simulink model "sm_trackV_roller4_IdlerArm_i2u0r3_ptcld"  (R2026a)
settings: Solver=ode23t  StopTime=14  AbsTol=1e-3  EnableMultiTasking=on
PostLoadFcn:
  | set_param([bdroot '/Track FL'],'popup_sense_roller','Actuator Torque')
  | set_param([bdroot '/Track FR'],'popup_sense_roller','Actuator Torque')
  | set_param([bdroot '/Track RL'],'popup_sense_roller','Actuator Torque')
  | set_param([bdroot '/Track RR'],'popup_sense_roller','Actuator Torque')
StartFcn:
  | tic
StopFcn:
  | Elapsed_Sim_Time = toc;
  | disp(['Elapsed Sim Time = ' num2str(Elapsed_Sim_Time)]);
undefined symbols (not defined in the file): Scene, X, Y, Z
libraries: sm_lib x9, fl_lib x8, nesl_utility x5, sm_trackV_lib_chain_underc_elem x4, simulink x4, sm_rollerV_lib_lower_frame_idlerArm_i2u0l3 x4, sm_excv_chassis_lib x3, sm_rollerV_lib_terrain_contact_r5 x3
(part 1 of 2)
Description:
  | Belt Track (Four), Roller Contact Point Cloud
  | Copyright 2024-2026 The MathWorks, Inc.
settings Model: Creator=smiller  LastModifiedBy=smiller
settings DataIOCC: SignalLoggingName=logsout_sm_trackV_roller4_IdlerArm_i2u0r3_ptcld
settings DebuggingCC: SubsystemReferenceDiagnosticForUnitTest=warning
settings SimscapeCC: SimscapeNominalValues="[{\"value\":\"1\",\"unit\":\"A\"},{\"value\":\"1\",\"unit\":\"bar\"},{\"value\":\"1\",\"unit\":\"cm^2\"},{\"value\":\"1\",\"unit\":\"cm^3/s\"},{\"value\":\"1\",\"unit\":\"kJ/kg\"},{\"value\":\"1\",\"unit\":\"kW\"},{\"value\":\"1\",\"unit\":\"l\"},{\"value\":\"1\",\"unit\":\"N\"},{\"value\":\"1\",\"unit\":\"N*m\"},{\"value\":\"1\",\"unit\":\"V\"}]"  SimscapeLogSimulationStatistics=on  SimscapeLogName=simlog_sm_trackV_roller4_IdlerArm_i2u0r3_ptcld  SimscapeLogLimitData=off
settings DiagnosticsConfigSet: SimMechanicsUnconnectedFramePorts=none  SimMechanicsConflictingReferenceFrames=none
settings ExplorerConfigSet: InternalSimMechanicsExplorerSettings="<ExplorerConfiguration><canonicalview>default</canonicalview><AnimationSetting><BasePlaybackSpeed>1.0</BasePlaybackSpeed><PlaybackSpeedFactor>4.0</PlaybackSpeedFactor></AnimationSetting><TilePanel><TileInfo><Tiles Columns=\"2\" Count=\"3\" Rows=\"2\"><Column Weight=\"0.5\"/><Column Weight=\"0.5\"/><Row Weight=\"0.4992\"/><Row Weight=\"0.5008\"/><Tile Height=\"2\" Width=\"1\" X=\"0\" Y=\"0\"/><Tile Height=\"1\" Width=\"1\" X=\"1\" Y=\"0\"/><Tile Height=\"1\" Width=\"1\" X=\"1\" Y=\"1\"/></Tiles></TileInfo><SceneInfo><SceneViewer><BGColor><R>1</R><G>1</G><B>1</B></BGColor><Camera><DoPerspective>on</DoPerspective><Position><X>8</X><Y>-4.69999999999999929</Y><Z>3.49999999999999956</Z></Position><Center><X>7.32379042217759135</X><Y>-4.02379042217759064</Y><Z>3.20762829527726279</Z></Center><Up><X>0</X><Y>0</Y><Z>1</Z></Up><ViewLimDist>1</ViewLimDist><YLim>0.466307658154998583</YLim><XLim>0.48985854998100864</XLim></Camera></SceneViewer><SceneViewer><BGColor><R>1</R><G>1</G><B>1</B></BGColor><Camera><DoPerspective>on</DoPerspective><Position><X>3.92771833623717702e-16</X><Y>-4</Y><Z>1.10000000000000053</Z></Position><Center><X>1.70727228698686394e-16</X><Y>-3</Y><Z>1.10000000000000053</Z></Center><Up><X>0</X><Y>0</Y><Z>1</Z></Up><ViewLimDist>1</ViewLimDist><YLim>0.466307658154998583</YLim><XLim>0.996493077701092966</XLim></Camera></SceneViewer><SceneViewer><BGColor><R>1</R><G>1</G><B>1</B></BGColor><Camera><DoPerspective>on</DoPerspective><Position><X>2.00000000000000089</X><Y>-2.52493193448249121e-16</Y><Z>9</Z></Position><Center><X>2.00000000000000089</X><Y>-2.52493193448249121e-16</Y><Z>8</Z></Center><Up><X>0</X><Y>1</Y><Z>0</Z></Up><ViewLimDist>1</ViewLimDist><YLim>0.466307658154998583</YLim><XLim>0.993092077435901444</XLim></Camera></SceneViewer></SceneInfo></TilePanel><MechEditorPanel><Cameras><Camera><Id>Camera1</Id><Value><Name>Track_CtrRear_AimFront</Name><NativeCamera><PositionTrackingFeature>Chassis.Camera_Frames.CamF_CtrRear_AimLF.R</PositionTrackingFeature><CenterTrackingFeature>Config.World_Frame.W</CenterTrackingFeature><UpVectorTrackingFeature>Config.World_Frame.W</UpVectorTrackingFeature><CenterTrackingOrigin>off</CenterTrackingOrigin><CenterTrackingDirection>+X</CenterTrackingDirection><UpVectorTrackingDirection>+Z</UpVectorTrackingDirection></NativeCamera></Value></Camera><Camera><Id>Camera2</Id><Value><Name>Track_Left_AimRight</Name><NativeCamera><PositionTrackingFeature>Chassis.Camera_Frames.CamF_Left_AimRight.R</PositionTrackingFeature><CenterTrackingFeature>Chassis.Camera_Frames.CamF_Left_AimRight.R</CenterTrackingFeature><UpVectorTrackingFeature>Config.World_Frame.W</UpVectorTrackingFeature><CenterTrackingOrigin>off</CenterTrackingOrigin><CenterTrackingDirection>+X</CenterTrackingDirection><UpVectorTrackingDirection>+Z</UpVectorTrackingDirection></NativeCamera></Value></Camera><Camera><Id>Camera3</Id><Value><Name>Track_Front_AimLR</Name><NativeCamera><PositionTrackingFeature>Chassis.Camera_Frames.CamF_Front_AimLR.R</PositionTrackingFeature><CenterTrackingFeature>Chassis.Camera_Frames.Transform_Front_AimLR.F</CenterTrackingFeature><UpVectorTrackingFeature>Config.World_Frame.W</UpVectorTrackingFeature><CenterTrackingOrigin>off</CenterTrackingOrigin><CenterTrackingDirection>+X</CenterTrackingDirection><UpVectorTrackingDirection>+Z</UpVectorTrackingDirection></NativeCamera></Value></Camera><Camera><Id>Camera4</Id><Value><Name>Track_Right_AimLeftTL</Name><NativeCamera><PositionTrackingFeature>Chassis.Camera_Frames.CamF_Right_AimLeftTL.R</PositionTrackingFeature><CenterTrackingFeature>Chassis.Camera_Frames.CamF_Right_AimLeftTL.R</CenterTrackingFeature><UpVectorTrackingFeature>Config.World_Frame.W</UpVectorTrackingFeature><CenterTrackingOrigin>off</CenterTrackingOrigin><CenterTrackingDirection>+X</CenterTrackingDirection><UpVectorTrackingDirection>+Z</UpVectorTrackingDirection></NativeCamera></Value></Camera><Camera><Id>Camera5</Id><Value><Name>Track_Right_AimLeftTR</Name><NativeCamera><PositionTrackingFeature>Chassis.Camera_Frames.CamF_Right_AimLeftTR.R</PositionTrackingFeature><CenterTrackingFeature>Chassis.Camera_Frames.CamF_Right_AimLeftTR.R</CenterTrackingFeature><UpVectorTrackingFeature>Config.World_Frame.W</UpVectorTrackingFeature><CenterTrackingOrigin>off</CenterTrackingOrigin><CenterTrackingDirection>+X</CenterTrackingDirection><UpVectorTrackingDirection>+Z</UpVectorTrackingDirection></NativeCamera></Value></Camera><Camera><Id>Camera6</Id><Value><Name>Track_FR_AimFront</Name><NativeCamera><PositionTrackingFeature>Chassis.Camera_Frames.CamF_FR_Aim_Front_R</PositionTrackingFeature><CenterTrackingFeature>Chassis.Camera_Frames.CamF_FR_Aim_Front_R</CenterTrackingFeature><UpVectorTrackingFeature>Config.W</UpVectorTrackingFeature><CenterTrackingOrigin>off</CenterTrackingOrigin><CenterTrackingDirection>+X</CenterTrackingDirection><UpVectorTrackingDirection>+Z</UpVectorTrackingDirection></NativeCamera></Value></Camera><Camera><Id>Camera7</Id><Value><Name>TrackIsoFR</Name><NativeCamera><PositionKeyframeSet><Keyframe><Time>0</Time><Value><X>7.6744465174951229</X><Y>-7.3378434494995588</Y><Z>0.83192924808838675</Z></Value></Keyframe><Keyframe><Time>4.8580359639439301</Time><Value><X>7.6744465174951229</X><Y>-7.3378434494995588</Y><Z>0.83192924808838675</Z></Value></Keyframe><Keyframe><Time>7.0422197385672698</Time><Value><X>8.4041500304882533</X><Y>-6.0478565656515233</Y><Z>1.2378387423585568</Z></Value></Keyframe><Keyframe><Time>12.78196840006439</Time><Value><X>20.29732183415512</X><Y>-9.1045432763174095</Y><Z>1.6217023498793322</Z></Value></Keyframe></PositionKeyframeSet><CenterKeyframeSet><Keyframe><Time>0</Time><Value><X>-3.9707986865367024</X><Y>13.1242688081241</Y><Z>1.8580696339996621</Z></Value></Keyframe><Keyframe><Time>4.8580359639439301</Time><Value><X>4.507312599752261</X><Y>-1.7728039312810333</Y><Z>1.1110065851169071</Z></Value></Keyframe><Keyframe><Time>7.0422197385672698</Time><Value><X>6.9754199629584264</X><Y>-2.3648388994835718</Y><Z>1.2924635728623486</Z></Value></Keyframe><Keyframe><Time>12.78196840006439</Time><Value><X>16.536524754348189</X><Y>-2.4963653739311518</Y><Z>1.9530913158644347</Z></Value></Keyframe></CenterKeyframeSet><UpVectorKeyframeSet><Keyframe><Time>0</Time><Value><X>0.036204453435340365</X><Y>-0.029489201528742272</Y><Z>0.99890921736894867</Z></Value></Keyframe><Keyframe><Time>4.8580359639439301</Time><Value><X>0.036204453435340372</X><Y>-0.029489201528742279</Y><Z>0.99890921736894867</Z></Value></Keyframe><Keyframe><Time>7.0422197385672698</Time><Value><X>0.015774113925201387</X><Y>-0.0087099802030477149</Y><Z>0.99983764360756966</Z></Value></Keyframe><Keyframe><Time>12.78196840006439</Time><Value><X>0.036204453435340372</X><Y>-0.029489201528742286</Y><Z>0.99890921736894867</Z></Value></Keyframe></UpVectorKeyframeSet></NativeCamera></Value></Camera><Camera><Id>Camera8</Id><Value><Name>Track_IsoFR_Big</Name><NativeCamera><PositionTrackingFeature>Chassis.Camera_Frames.CamF_FR_AimCtr_Big.R</PositionTrackingFeature><CenterTrackingFeature>Chassis.Camera_Frames.CamF_FR_AimCtr_Big.R</CenterTrackingFeature><UpVectorTrackingFeature>Config.W.frame</UpVectorTrackingFeature><CenterTrackingOrigin>off</CenterTrackingOrigin><CenterTrackingDirection>+X</CenterTrackingDirection><UpVectorTrackingDirection>+Z</UpVectorTrackingDirection></NativeCamera></Value></Camera><Camera><Id>Camera9</Id><Value><Name>Track_Top_FixO</Name><NativeCamera><PositionTrackingFeature>Chassis.Camera_Frames.CamF_Top.R</PositionTrackingFeature><CenterTrackingFeature>Config.W</CenterTrackingFeature><UpVectorTrackingFeature>Config.W</UpVectorTrackingFeature><CenterTrackingOrigin>off</CenterTrackingOrigin><CenterTrackingDirection>-Z</CenterTrackingDirection><UpVectorTrackingDirection>+Y</UpVectorTrackingDirection></NativeCamera></Value></Camera><Camera><Id>Camera10</Id><Value><Name>Track_Terrain_Steer</Name><NativeCamera><PositionKeyframeSet><Keyframe><Time>1.954306185234983</Time><Value><X>6.8114446186923496</X><Y>-5.3171553607278206</Y><Z>2.3434891046120194</Z></Value></Keyframe><Keyframe><Time>3.2620190833091063</Time><Value><X>8.6993949048857981</X><Y>-5.3317331728841273</Y><Z>2.4343360662333233</Z></Value></Keyframe><Keyframe><Time>5.0400013056141875</Time><Value><X>10.892348868797249</X><Y>-5.3777629823446311</Y><Z>2.9548739629979583</Z></Value></Keyframe><Keyframe><Time>6.4399956757078574</Time><Value><X>12.590773161836934</X><Y>-5.02192612890686</Y><Z>3.4550574594673802</Z></Value></Keyframe><Keyframe><Time>8.274080048576554</Time><Value><X>14.467163111987707</X><Y>-3.5325878594240057</Y><Z>3.6687375492730663</Z></Value></Keyframe><Keyframe><Time>10.611771973115053</Time><Value><X>16.092056497155664</X><Y>-0.19034994331009364</Y><Z>3.5642210119966649</Z></Value></Keyframe><Keyframe><Time>12.781922870204893</Time><Value><X>16.438502065245114</X><Y>2.6045222313399137</Y><Z>3.7512090554216835</Z></Value></Keyframe><Keyframe><Time>14</Time><Value><X>15.821419267246833</X><Y>4.405488260701441</Y><Z>3.6561806172412985</Z></Value></Keyframe></PositionKeyframeSet><CenterKeyframeSet><Keyframe><Time>1.954306185234983</Time><Value><X>3.8269446610796178</X><Y>-1.4237791566024609</Y><Z>1.4146779468278596</Z></Value></Keyframe><Keyframe><Time>3.2620190833091063</Time><Value><X>5.6599243323637811</X><Y>-1.3666460332407318</Y><Z>1.4884174126531708</Z></Value></Keyframe><Keyframe><Time>5.0400013056141875</Time><Value><X>7.9655341663497534</X><Y>-1.5596390492794066</Y><Z>2.0440151286844124</Z></Value></Keyframe><Keyframe><Time>6.4399956757078574</Time><Value><X>8.8172775775206471</X><Y>-0.099279748271351664</Y><Z>2.280701670444107</Z></Value></Keyframe><Keyframe><Time>8.274080048576554</Time><Value><X>11.140862936281749</X><Y>0.80667772469433485</Y><Z>2.633554181468174</Z></Value></Keyframe><Keyframe><Time>10.611771973115053</Time><Value><X>12.246653975093967</X><Y>4.8261013508136488</Y><Z>2.3674869461938366</Z></Value></Keyframe><Keyframe><Time>12.781922870204893</Time><Value><X>13.419912109075547</X><Y>6.5423699352357101</Y><Z>2.8117886929204419</Z></Value></Keyframe><Keyframe><Time>14</Time><Value><X>13.045484539267546</X><Y>8.0267844133623925</Y><Z>2.7922773888123493</Z></Value></Keyframe></CenterKeyframeSet><UpVectorKeyframeSet><Keyframe><Time>1.954306185234983</Time><Value><X>-0.1264530356370476</X><Y>0.13743109156705063</Y><Z>0.98240639495519599</Z></Value></Keyframe><Keyframe><Time>3.2620190833091063</Time><Value><X>-0.1264530356370476</X><Y>0.13743109156705063</Y><Z>0.98240639495519599</Z></Value></Keyframe><Keyframe><Time>5.0400013056141875</Time><Value><X>-0.12645303563704768</X><Y>0.13743109156705072</Y><Z>0.98240639495519599</Z></Value></Keyframe><Keyframe><Time>6.4399956757078574</Time><Value><X>-0.12645303563704768</X><Y>0.13743109156705072</Y><Z>0.98240639495519599</Z></Value></Keyframe><Keyframe><Time>8.274080048576554</Time><Value><X>-0.12645303563704768</X><Y>0.13743109156705069</Y><Z>0.98240639495519611</Z></Value></Keyframe><Keyframe><Time>10.611771973115053</Time><Value><X>-0.12645303563704768</X><Y>0.13743109156705069</Y><Z>0.98240639495519599</Z></Value></Keyframe><Keyframe><Time>12.781922870204893</Time><Value><X>-0.12645303563704771</X><Y>0.13743109156705072</Y><Z>0.98240639495519599</Z></Value></Keyframe><Keyframe><Time>14</Time><Value><X>-0.12645303563704774</X><Y>0.13743109156705072</Y><Z>0.98240639495519588</Z></Value></Keyframe></UpVectorKeyframeSet></NativeCamera></Value></Camera></Cameras><GfxPanelCameraMap><MapElement CameraMLId=\"Camera8\" GfxPanelIndex=\"0\"/><MapElement CameraMLId=\"Camera5\" GfxPanelIndex=\"1\"/><MapElement CameraMLId=\"Camera9\" GfxPanelIndex=\"2\"/></GfxPanelCameraMap><VideoCreator><PlaybackSpeedRatio>0.5</PlaybackSpeedRatio><FrameRate>30</FrameRate><VideoFormat>MPEG-4</VideoFormat><FrameSize>auto</FrameSize></VideoCreator></MechEditorPanel></ExplorerConfiguration>"

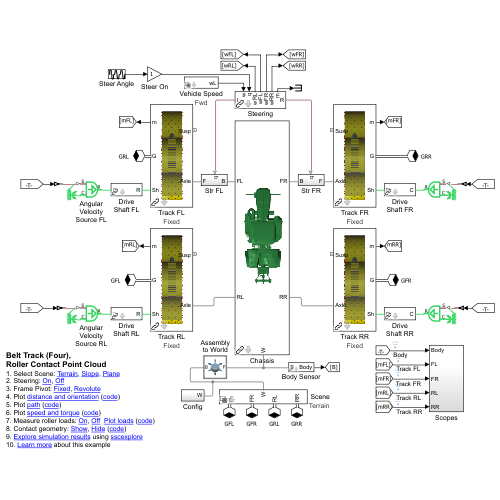
[thumbnail: Simulink's stored preview of the top-level diagram]
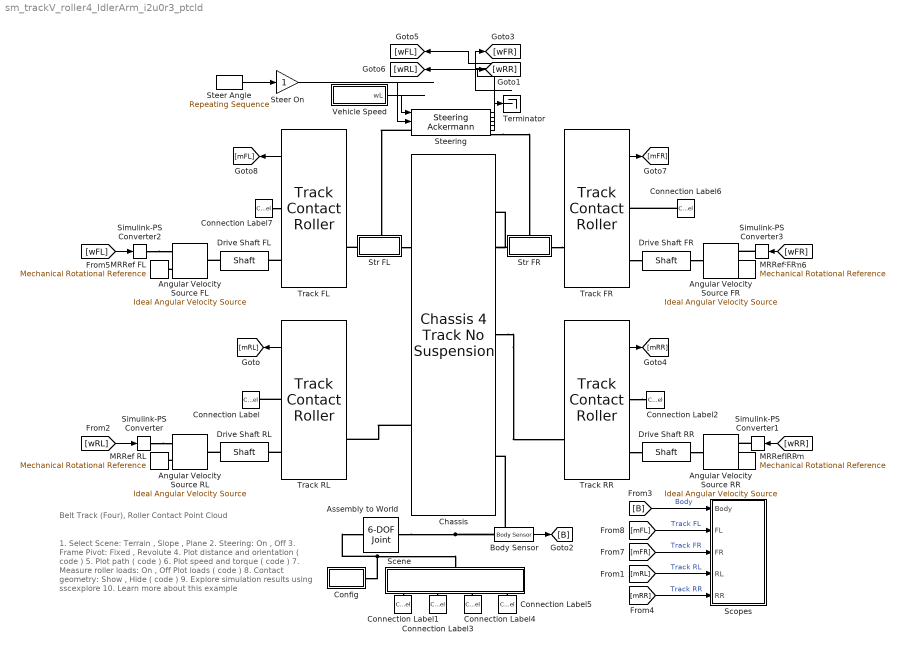
== system sm_trackV_roller4_IdlerArm_i2u0r3_ptcld ==
  note: 1. Select Scene: Terrain , Slope , Plane
      | 2. Steering: On , Off
      | 3. Frame Pivot: Fixed , Revolute
      | 4. Plot distance and orientation ( code )
      | 5. Plot path ( code )
      | 6. Plot speed and torque ( code )
      | 7. Measure roller loads: On , Off Plot loads ( code )
      | 8. Contact geometry: Show , Hide ( code )
      | 9. Explore simulation results using sscexplore
      | 10. Learn more about this example
  note: Belt Track (Four),
      | Roller Contact Point Cloud
  Angular Velocity Source FL : fl_lib/Mechanical/Mechanical Sources/Ideal Angular Velocity Source
  Angular Velocity Source FR : fl_lib/Mechanical/Mechanical Sources/Ideal Angular Velocity Source
  Angular Velocity Source RL : fl_lib/Mechanical/Mechanical Sources/Ideal Angular Velocity Source
  Angular Velocity Source RR : fl_lib/Mechanical/Mechanical Sources/Ideal Angular Velocity Source
  Assembly to World : sm_lib/Joints/6-DOF Joint  JointMode=Normal  CompositeWrenchDir=FollowerOnBase  CompositeWrenchFrame=BaseFrame  SenseConstraintForce=off  SenseConstraintTorque=off  SenseTotalForce=off  SenseTotalTorque=off  PxPositionTargetSpecify=on  PxPositionTargetPriority=High  PxPositionTargetValue=0  PxPositionTargetValueUnits=m  PxVelocityTargetSpecify=off  PxVelocityTargetPriority=High  PxVelocityTargetValue=0  PxVelocityTargetValueUnits=m/s  PxEquilibriumPosition=0  PxEquilibriumPositionUnits=m  PxSpringStiffness=0  PxSpringStiffnessUnits=N/m  PxDampingCoefficient=0  PxDampingCoefficientUnits=N/(m/s)  PxLowerLimitSpecify=off  PxLowerLimitBound=-1  PxLowerLimitBoundUnits=m  PxLowerLimitStiffness=1e6  PxLowerLimitStiffnessUnits=N/m  PxLowerLimitDamping=1e3  PxLowerLimitDampingUnits=N/(m/s)  PxLowerLimitTransitionRegionWidth=1e-4  PxLowerLimitTransitionRegionWidthUnits=m  PxUpperLimitSpecify=off  PxUpperLimitBound=1  PxUpperLimitBoundUnits=m  PxUpperLimitStiffness=1e6  PxUpperLimitStiffnessUnits=N/m  PxUpperLimitDamping=1e3  PxUpperLimitDampingUnits=N/(m/s)  PxUpperLimitTransitionRegionWidth=1e-4  PxUpperLimitTransitionRegionWidthUnits=m  PxTorqueActuationMode=NoTorque  PxMotionActuationMode=ComputedMotion  PxSensePosition=off  PxSenseVelocity=off  PxSenseAcceleration=off  PxSenseTorqueForce=off  PxSenseLowerLimitTorqueForce=off  PxSenseUpperLimitTorqueForce=off  PyPositionTargetSpecify=on  PyPositionTargetPriority=High  PyPositionTargetValue=0  PyPositionTargetValueUnits=m  PyVelocityTargetSpecify=off  PyVelocityTargetPriority=High  PyVelocityTargetValue=0  PyVelocityTargetValueUnits=m/s  PyEquilibriumPosition=0  PyEquilibriumPositionUnits=m  PySpringStiffness=0  PySpringStiffnessUnits=N/m  PyDampingCoefficient=0  PyDampingCoefficientUnits=N/(m/s)  PyLowerLimitSpecify=off  PyLowerLimitBound=-1  PyLowerLimitBoundUnits=m  PyLowerLimitStiffness=1e6  PyLowerLimitStiffnessUnits=N/m  PyLowerLimitDamping=1e3  PyLowerLimitDampingUnits=N/(m/s)  PyLowerLimitTransitionRegionWidth=1e-4  PyLowerLimitTransitionRegionWidthUnits=m  PyUpperLimitSpecify=off  PyUpperLimitBound=1  PyUpperLimitBoundUnits=m  PyUpperLimitStiffness=1e6  PyUpperLimitStiffnessUnits=N/m  PyUpperLimitDamping=1e3  PyUpperLimitDampingUnits=N/(m/s)  PyUpperLimitTransitionRegionWidth=1e-4  PyUpperLimitTransitionRegionWidthUnits=m  PyTorqueActuationMode=NoTorque  PyMotionActuationMode=ComputedMotion  PySensePosition=off  PySenseVelocity=off  PySenseAcceleration=off  PySenseTorqueForce=off  PySenseLowerLimitTorqueForce=off  PySenseUpperLimitTorqueForce=off  PzPositionTargetSpecify=on  PzPositionTargetPriority=High  PzPositionTargetValue=1.5  PzPositionTargetValueUnits=m  PzVelocityTargetSpecify=off  PzVelocityTargetPriority=High  PzVelocityTargetValue=0  PzVelocityTargetValueUnits=m/s  PzEquilibriumPosition=0  PzEquilibriumPositionUnits=m  PzSpringStiffness=0  PzSpringStiffnessUnits=N/m  PzDampingCoefficient=0  PzDampingCoefficientUnits=N/(m/s)  PzLowerLimitSpecify=off  PzLowerLimitBound=-1  PzLowerLimitBoundUnits=m  PzLowerLimitStiffness=1e6  PzLowerLimitStiffnessUnits=N/m  PzLowerLimitDamping=1e3  PzLowerLimitDampingUnits=N/(m/s)  PzLowerLimitTransitionRegionWidth=1e-4  PzLowerLimitTransitionRegionWidthUnits=m  PzUpperLimitSpecify=off  PzUpperLimitBound=1  PzUpperLimitBoundUnits=m  PzUpperLimitStiffness=1e6  PzUpperLimitStiffnessUnits=N/m  PzUpperLimitDamping=1e3  PzUpperLimitDampingUnits=N/(m/s)  PzUpperLimitTransitionRegionWidth=1e-4  PzUpperLimitTransitionRegionWidthUnits=m  PzTorqueActuationMode=NoTorque  PzMotionActuationMode=ComputedMotion  PzSensePosition=off  PzSenseVelocity=off  PzSenseAcceleration=off  PzSenseTorqueForce=off  PzSenseLowerLimitTorqueForce=off  PzSenseUpperLimitTorqueForce=off  SphPositionTargetSpecify=off  SphPositionTargetPriority=High  SphPositionTargetRotationMethod=StandardAxis  SphPositionTargetFollAlignAxisA=+X  SphPositionTargetBaseAlignAxisA=+Y  SphPositionTargetFollAlignAxisB=+Y  SphPositionTargetBaseAlignAxisB=+Z  SphPositionTargetRotationStandardAxis=+Z  SphPositionTargetRotationAngle=180  SphPositionTargetRotationAngleUnits=deg  SphPositionTargetRotationArbitraryAxis=[0 0 1]  SphPositionTargetRotationSequenceAxes=FollowerAxes  SphPositionTargetRotationSequence=XYX  SphPositionTargetRotationSequenceAngles=[0 0 0]  SphPositionTargetRotationSequenceAnglesUnits=deg  SphPositionTargetRotationMatrix=[1 0 0; 0 1 0; 0 0 1]  SphPositionTargetQuaternion=[1 0 0 0]  SphVelocityTargetSpecify=off  SphVelocityTargetPriority=High  SphVelocityTargetValue=[0 0 0]  SphVelocityTargetValueUnits=deg/s  SphVelocityTargetInFollowerFrame=on  SphEqPosRotationMethod=None  SphEqPosFollAlignAxisA=+X  SphEqPosBaseAlignAxisA=+Y  SphEqPosFollAlignAxisB=+Y  SphEqPosBaseAlignAxisB=+Z  SphEqPosRotationStandardAxis=+Z  SphEqPosRotationAngle=0.0  SphEqPosRotationAngleUnits=deg  SphEqPosRotationArbitraryAxis=[0 0 1]  SphEqPosRotationSequenceAxes=FollowerAxes  SphEqPosRotationSequence=XYX  SphEqPosRotationSequenceAngles=[0 0 0]  SphEqPosRotationSequenceAnglesUnits=deg  SphEqPosRotationMatrix=[1 0 0; 0 1 0; 0 0 1]  SphEqPosQuaternion=[1 0 0 0]  SphSpringStiffness=0  SphSpringStiffnessUnits=N*m/deg  SphDampingCoefficient=0  SphDampingCoefficientUnits=N*m/(deg/s)  SphLowerLimitSpecify=off  SphLowerLimitBound=15  SphLowerLimitBoundUnits=deg  SphLowerLimitStiffness=1e4  SphLowerLimitStiffnessUnits=N*m/deg  SphLowerLimitDamping=10  SphLowerLimitDampingUnits=N*m/(deg/s)  SphLowerLimitTransitionRegionWidth=0.1  SphLowerLimitTransitionRegionWidthUnits=deg  SphUpperLimitSpecify=off  SphUpperLimitBound=45  SphUpperLimitBoundUnits=deg  SphUpperLimitStiffness=1e4  SphUpperLimitStiffnessUnits=N*m/deg  SphUpperLimitDamping=10  SphUpperLimitDampingUnits=N*m/(deg/s)  SphUpperLimitTransitionRegionWidth=0.1  SphUpperLimitTransitionRegionWidthUnits=deg  SphTorqueActuationMode=NoTorque  SphActuateTorqueX=off  SphActuateTorqueY=off  SphActuateTorqueZ=off  SphActuateTorque=off  SphActuationFrame=BaseFrame  SphSensePosition=off  SphSenseVelocityX=off  SphSenseVelocityY=off  SphSenseVelocityZ=off  SphSenseVelocity=off  SphSenseAccelerationX=off  SphSenseAccelerationY=off  SphSenseAccelerationZ=off  SphSenseAcceleration=off  SphSenseLowerLimitTorqueMag=off  SphSenseUpperLimitTorqueMag=off  SphSensingFrame=BaseFrame
  Body Sensor : sm_excv_chassis_lib/Body Sensor  offset_body_sensor=[0 0 0]
  Chassis : sm_excv_chassis_lib/Chassis 4 Track No Suspension  popup_chassis_geo=CAD Shell
  Config : Subsystem
  Connection Label : ConnectionLabel  Label=GFL
  Connection Label1 : ConnectionLabel  Label=GFL
  Connection Label2 : ConnectionLabel  Label=GFR
  Connection Label3 : ConnectionLabel  Label=GFR
  Connection Label4 : ConnectionLabel  Label=GRL
  Connection Label5 : ConnectionLabel  Label=GRR
  Connection Label6 : ConnectionLabel  Label=GRR
  Connection Label7 : ConnectionLabel  Label=GRL
  Drive Shaft FL : sm_trackV_lib_chain_underc_elem/Shaft  k_shaft=Excv.Drive.Shaft.k  b_shaft=Excv.Drive.Shaft.b
  Drive Shaft FR : sm_trackV_lib_chain_underc_elem/Shaft  k_shaft=Excv.Drive.Shaft.k  b_shaft=Excv.Drive.Shaft.b
  Drive Shaft RL : sm_trackV_lib_chain_underc_elem/Shaft  k_shaft=Excv.Drive.Shaft.k  b_shaft=Excv.Drive.Shaft.b
  Drive Shaft RR : sm_trackV_lib_chain_underc_elem/Shaft  k_shaft=Excv.Drive.Shaft.k  b_shaft=Excv.Drive.Shaft.b
  MRRef FL : fl_lib/Mechanical/Rotational Elements/Mechanical Rotational Reference
  MRRef FR : fl_lib/Mechanical/Rotational Elements/Mechanical Rotational Reference
  MRRef RL : fl_lib/Mechanical/Rotational Elements/Mechanical Rotational Reference
  MRRef RR : fl_lib/Mechanical/Rotational Elements/Mechanical Rotational Reference
  Scene : Subsystem  Variant=on  VariantControlMode=label  VariantControl=Terrain  LabelModeActiveChoice=Terrain
      settings: AttributesFormatString=%<LabelModeActiveChoice>
      mask Display: disp(' ')
  Scopes : Subsystem
  Simulink-PS Converter{,1..3} (4 alike) : nesl_utility/Simulink-PS Converter  PhysicalDomain=network_engine_domain  SubClassName=ps_input  LeftPortType=input  RightPortType=output  PseudoPeriodic=off  Frequencies=[]  NoiseDistribution=none  NoiseParameters=[]  Unit=1  AffineConversion=off  FilteringAndDerivatives=provide  SimscapeFilterOrder=1  InputFilterTimeConstant=0.001  UdotUserProvided=0
  Steer Angle : simulink/Sources/Repeating Sequence  rep_seq_t="[0 3  5  14 16 18  20  29 31 36]"  rep_seq_y="[0 0 20 20  0   0 -20 -20  0   0]*pi/180"
  Steer On : Gain
  Steering : sm_excv_chassis_lib/Steering Ackermann  yTrack=Trac.Chassis.Front.TrackSepCtr  steerRatio=1  tcSteer=0.1  wheelbase=Trac.Chassis.AxleSeparation
  Str FL : Subsystem
      settings: PortSchema="{\"entries\":[{\"content\":{\"sides\":[{\"content\":{\"connectorIds\":[\"LConn1\"]},\"type\":\"ConnectorPlacement.EquallySpacedRectSide\",\"uuid\":\"c7c7e178-8ee1-427d-9e3f-0887a6c2686c\"},{\"content\":{\"connectorIds\":[\"RConn1\"],\"side\":\"RIGHT\"},\"type\":\"ConnectorPlacement.EquallySpacedRectSide\",\"uuid\":\"0bc250c9-893f-4ff8-8fb1-de52c2b7a8cd\"},{\"content\":{\"connectorIds\":[\"LConn2\"],\"side\":\"TOP\"},\"type\":\"ConnectorPlacement.EquallySpacedRectSide\",\"uuid\":\"31ffd3a3-da84-490a-ac6f-43ff5d5145cd\"}]},\"type\":\"ConnectorPlacement.EquallySpacedConnector\",\"uuid\":\"2f775820-965f-444f-9db7-4d7e95d78bbe\"}],\"packageUris\":[\"http://schema.mathworks.com/mf0/Connector/R2020b\"],\"version\":\"1.0\"}"
  Str FR : Subsystem
      settings: PortSchema="{\"entries\":[{\"content\":{\"sides\":[{\"content\":{\"connectorIds\":[\"LConn1\"]},\"type\":\"ConnectorPlacement.EquallySpacedRectSide\",\"uuid\":\"c7c7e178-8ee1-427d-9e3f-0887a6c2686c\"},{\"content\":{\"connectorIds\":[\"RConn1\"],\"side\":\"RIGHT\"},\"type\":\"ConnectorPlacement.EquallySpacedRectSide\",\"uuid\":\"0bc250c9-893f-4ff8-8fb1-de52c2b7a8cd\"},{\"content\":{\"connectorIds\":[\"LConn2\"],\"side\":\"TOP\"},\"type\":\"ConnectorPlacement.EquallySpacedRectSide\",\"uuid\":\"31ffd3a3-da84-490a-ac6f-43ff5d5145cd\"}]},\"type\":\"ConnectorPlacement.EquallySpacedConnector\",\"uuid\":\"2f775820-965f-444f-9db7-4d7e95d78bbe\"}],\"packageUris\":[\"http://schema.mathworks.com/mf0/Connector/R2020b\"],\"version\":\"1.0\"}"
  Terminator : Terminator
  Track FL : sm_rollerV_lib_lower_frame_idlerArm_i2u0l3/Track Contact Roller  sprk_wid_roll=Trac.Sprocket.Roller.wid  sprk_rad_roll=Trac.Sprocket.Roller.rad  sprk_clr=Trac.Sprocket.Roller.clr  sprk_opc=Trac.Sprocket.Roller.opc  sprk_rad_pitch=Trac.Sprocket.Spoke.pitch_rad  sprk_spoke_rad=Trac.Sprocket.Spoke.rad  sprk_spoke_num=Trac.Sprocket.nSpokes  sprk_spoke_len=Trac.Sprocket.Spoke.len  sprk_rim_spoke_xc=Trac.Sprocket.Rim.spoke_xc  sprk_rim_ir=Trac.Sprocket.Rim.rad_inner  sprk_rim_thk=Trac.Sprocket.Rim.thk  idlerR_rad=Trac.IdlerR.rad  idlerF_rad=Trac.IdlerF.rad  idlerR_total_len=Trac.IdlerR.len_total  idlerF_total_len=Trac.IdlerF.len_total  idlerR_avg_rho=Trac.IdlerR.rho_avg  idlerF_avg_rho=Trac.IdlerF.rho_avg  idlerR_clr=Trac.IdlerR.clr  idlerF_clr=Trac.IdlerF.clr  idlerR_opc=Trac.IdlerR.opc  idlerF_opc=Trac.IdlerF.opc  idlerR_contgeo_ptcld=Trac.IdlerR.ground_contact.ptcld.pts  idlerF_contgeo_ptcld=Trac.IdlerF.ground_contact.ptcld.pts  idlerR_contgeo_rad=Trac.IdlerR.ground_contact.ptcld.rad  idlerF_contgeo_rad=Trac.IdlerF.ground_contact.ptcld.rad  idlerR_contgeo_clr=Trac.IdlerR.belt_contact.clr  idlerF_contgeo_clr=Trac.IdlerF.belt_contact.clr  idlerR_contgeo_opc=Trac.IdlerR.belt_contact.opc  idlerF_contgeo_opc=Trac.IdlerF.belt_contact.opc  arm_idlerc=Trac.IdlerArm.Pivot_to_Idler  arm_tens_x=Trac.IdlerArm.Pivot_to_TensionerX  arm_tens_y=Trac.IdlerArm.Pivot_to_TensionerY  arm_wid=Trac.IdlerArm.wid  arm_thk=Trac.IdlerArm.thk  arm_rho=Trac.IdlerArm.rho  arm_clr=Trac.IdlerArm.clr  arm_opc=Trac.IdlerArm.opc  roller_lower_rad=Trac.Roller.Lower.rad  roller_lower_len=Trac.Roller.Lower.len  roller_lower_rho=Trac.Roller.Lower.rho  roller_lower_clr=Trac.Roller.Lower.clr  roller_lower_opc=Trac.Roller.Lower.opc  roller_lower_contgeo_ptcld=Trac.Roller.Lower.ground_contact.ptcld.pts  roller_lower_contgeo_rad=Trac.Roller.Lower.ground_contact.ptcld.rad  roller_lower_contgeo_clr=Trac.Roller.Lower.belt_contact.clr  roller_lower_contgeo_opc=Trac.Roller.Lower.belt_contact.opc  tensioner_cyl_len=Trac.IdlerF.Tensioner.cyl.len  tensioner_cyl_rad=Trac.IdlerF.Tensioner.cyl.rad  tensioner_cyl_rho=Trac.IdlerF.Tensioner.cyl.rho  tensioner_cyl_clr=Trac.IdlerF.Tensioner.cyl.clr  tensioner_cyl_opc=Trac.IdlerF.Tensioner.cyl.opc  tensioner_pist_len=Trac.IdlerF.Tensioner.piston.len  tensioner_pist_rad=Trac.IdlerF.Tensioner.piston.rad  tensioner_pist_rho=Trac.IdlerF.Tensioner.piston.rho  tensioner_pist_clr=Trac.IdlerF.Tensioner.piston.clr  tensioner_pist_opc=Trac.IdlerF.Tensioner.piston.opc  tensioner_br_len=Trac.IdlerF.Tensioner.bracket.len  tensioner_br_width=Trac.IdlerF.Tensioner.bracket.wid  tensioner_br_height=Trac.IdlerF.Tensioner.bracket.height  tensioner_br_thk=Trac.IdlerF.Tensioner.bracket.thk  tensioner_br_rho=Trac.IdlerF.Tensioner.bracket.rho  tensioner_br_clr=Trac.IdlerF.Tensioner.bracket.clr  tensioner_br_opc=Trac.IdlerF.Tensioner.bracket.opc  tensioner_eqpos=Trac.IdlerF.Tensioner.xeq  tensioner_x0=Trac.IdlerF.Tensioner.x0  tensioner_k=Trac.IdlerF.Tensioner.K  tensioner_b=Trac.IdlerF.Tensioner.B  popup_leftOrRight=Left  popup_trackFrame=Fixed  roller_lower_x=Trac.Frame.SprkOffLon.Lower  idlerFix_x=Trac.Frame.SprkOffLon.IdlerR  idlerArm_x=Trac.Frame.SprkOffLon.IdlerArm  tensionC_x=Trac.Frame.SprkOffLon.TensionC  frame_pivot_x=Trac.Frame.SprkOffLon.PivotFra  axle_x=Trac.Frame.SprkOffLon.Axle  roller_lower_y=Trac.Frame.SprkOffVer.Lower  idlerFix_y=Trac.Frame.SprkOffVer.IdlerR  tensionC_y=Trac.Frame.SprkOffVer.TensionC  frame_pivot_y=Trac.Frame.SprkOffVer.PivotFra  axle_y=Trac.Frame.SprkOffVer.Axle  idlerArm_y=Trac.Frame.SprkOffVer.IdlerArm  frame_mass=Trac.Frame.TrackFrame.Mass  frame_cg_offset=Trac.Frame.TrackFrame.CG  frame_moi=Trac.Frame.TrackFrame.MOI  frame_poi=Trac.Frame.TrackFrame.POI  frame_roller_cg_offset=Trac.Frame.SprkFrame.CG  frame_roller_mass=Trac.Frame.SprkFrame.Mass  frame_roller_moi=Trac.Frame.SprkFrame.MOI  frame_roller_poi=Trac.Frame.SprkFrame.POI  frame_susp_offset=Trac.Frame.SuspOffset  roller_frame_pivot_range=Trac.Frame.PivotFra.Range  roller_frame_pivot_k=Trac.Frame.PivotFra.LimitK  roller_frame_pivot_b=Trac.Frame.PivotFra.LimitB  roller_frame_pivot_tw=Trac.Frame.PivotFra.LimitTW  sprk_rolling_rad=Trac.Sprocket.ground_contact.rolling_radius  roller_lower_rolling_rad=Trac.Roller.Lower.ground_contact.rolling_radius  idlerF_rolling_rad=Trac.IdlerF.ground_contact.rolling_radius  idlerR_rolling_rad=Trac.IdlerR.ground_contact.rolling_radius  rolling_cyl_len=Trac.Belt.w  accent_vis_lext=1e-3  roller_lower_cyl_clr=Trac.Roller.Lower.clr  roller_lower_cyl_opc=Trac.Roller.Lower.opc  idlerR_rollvervis_clr=Trac.IdlerR.clr  idlerF_rollvervis_clr=Trac.IdlerF.clr  idlerR_rollervis_opc=Trac.IdlerR.opc  idlerF_rollervis_opc=Trac.IdlerF.opc  accMn=0.65  accMx=0.75  acc_clr=[0.8 0.8 0.8]  acc_opc=1  track_m=Trac.Vis.Track.m  track_cg_offset=Trac.Vis.Track.cg  track_moi=Trac.Vis.Track.moi  track_poi=Trac.Vis.Track.poi  track_xc=Trac.Vis.Track.track_xc  track_clr=Trac.Vis.Track.clr  track_opc=Trac.Vis.Track.opc  popup_sense_roller=Actuator Torque
      settings: AttributesFormatString=%<popup_trackFrame>
  Track FR : sm_rollerV_lib_lower_frame_idlerArm_i2u0l3/Track Contact Roller  sprk_wid_roll=Trac.Sprocket.Roller.wid  sprk_rad_roll=Trac.Sprocket.Roller.rad  sprk_clr=Trac.Sprocket.Roller.clr  sprk_opc=Trac.Sprocket.Roller.opc  sprk_rad_pitch=Trac.Sprocket.Spoke.pitch_rad  sprk_spoke_rad=Trac.Sprocket.Spoke.rad  sprk_spoke_num=Trac.Sprocket.nSpokes  sprk_spoke_len=Trac.Sprocket.Spoke.len  sprk_rim_spoke_xc=Trac.Sprocket.Rim.spoke_xc  sprk_rim_ir=Trac.Sprocket.Rim.rad_inner  sprk_rim_thk=Trac.Sprocket.Rim.thk  idlerR_rad=Trac.IdlerR.rad  idlerF_rad=Trac.IdlerF.rad  idlerR_total_len=Trac.IdlerR.len_total  idlerF_total_len=Trac.IdlerF.len_total  idlerR_avg_rho=Trac.IdlerR.rho_avg  idlerF_avg_rho=Trac.IdlerF.rho_avg  idlerR_clr=Trac.IdlerR.clr  idlerF_clr=Trac.IdlerF.clr  idlerR_opc=Trac.IdlerR.opc  idlerF_opc=Trac.IdlerF.opc  idlerR_contgeo_ptcld=Trac.IdlerR.ground_contact.ptcld.pts  idlerF_contgeo_ptcld=Trac.IdlerF.ground_contact.ptcld.pts  idlerR_contgeo_rad=Trac.IdlerR.ground_contact.ptcld.rad  idlerF_contgeo_rad=Trac.IdlerF.ground_contact.ptcld.rad  idlerR_contgeo_clr=Trac.IdlerR.belt_contact.clr  idlerF_contgeo_clr=Trac.IdlerF.belt_contact.clr  idlerR_contgeo_opc=Trac.IdlerR.belt_contact.opc  idlerF_contgeo_opc=Trac.IdlerF.belt_contact.opc  arm_idlerc=Trac.IdlerArm.Pivot_to_Idler  arm_tens_x=Trac.IdlerArm.Pivot_to_TensionerX  arm_tens_y=Trac.IdlerArm.Pivot_to_TensionerY  arm_wid=Trac.IdlerArm.wid  arm_thk=Trac.IdlerArm.thk  arm_rho=Trac.IdlerArm.rho  arm_clr=Trac.IdlerArm.clr  arm_opc=Trac.IdlerArm.opc  roller_lower_rad=Trac.Roller.Lower.rad  roller_lower_len=Trac.Roller.Lower.len  roller_lower_rho=Trac.Roller.Lower.rho  roller_lower_clr=Trac.Roller.Lower.clr  roller_lower_opc=Trac.Roller.Lower.opc  roller_lower_contgeo_ptcld=Trac.Roller.Lower.ground_contact.ptcld.pts  roller_lower_contgeo_rad=Trac.Roller.Lower.ground_contact.ptcld.rad  roller_lower_contgeo_clr=Trac.Roller.Lower.belt_contact.clr  roller_lower_contgeo_opc=Trac.Roller.Lower.belt_contact.opc  tensioner_cyl_len=Trac.IdlerF.Tensioner.cyl.len  tensioner_cyl_rad=Trac.IdlerF.Tensioner.cyl.rad  tensioner_cyl_rho=Trac.IdlerF.Tensioner.cyl.rho  tensioner_cyl_clr=Trac.IdlerF.Tensioner.cyl.clr  tensioner_cyl_opc=Trac.IdlerF.Tensioner.cyl.opc  tensioner_pist_len=Trac.IdlerF.Tensioner.piston.len  tensioner_pist_rad=Trac.IdlerF.Tensioner.piston.rad  tensioner_pist_rho=Trac.IdlerF.Tensioner.piston.rho  tensioner_pist_clr=Trac.IdlerF.Tensioner.piston.clr  tensioner_pist_opc=Trac.IdlerF.Tensioner.piston.opc  tensioner_br_len=Trac.IdlerF.Tensioner.bracket.len  tensioner_br_width=Trac.IdlerF.Tensioner.bracket.wid  tensioner_br_height=Trac.IdlerF.Tensioner.bracket.height  tensioner_br_thk=Trac.IdlerF.Tensioner.bracket.thk  tensioner_br_rho=Trac.IdlerF.Tensioner.bracket.rho  tensioner_br_clr=Trac.IdlerF.Tensioner.bracket.clr  tensioner_br_opc=Trac.IdlerF.Tensioner.bracket.opc  tensioner_eqpos=Trac.IdlerF.Tensioner.xeq  tensioner_x0=Trac.IdlerF.Tensioner.x0  tensioner_k=Trac.IdlerF.Tensioner.K  tensioner_b=Trac.IdlerF.Tensioner.B  popup_leftOrRight=Right  popup_trackFrame=Fixed  roller_lower_x=Trac.Frame.SprkOffLon.Lower  idlerFix_x=Trac.Frame.SprkOffLon.IdlerR  idlerArm_x=Trac.Frame.SprkOffLon.IdlerArm  tensionC_x=Trac.Frame.SprkOffLon.TensionC  frame_pivot_x=Trac.Frame.SprkOffLon.PivotFra  axle_x=Trac.Frame.SprkOffLon.Axle  roller_lower_y=Trac.Frame.SprkOffVer.Lower  idlerFix_y=Trac.Frame.SprkOffVer.IdlerR  tensionC_y=Trac.Frame.SprkOffVer.TensionC  frame_pivot_y=Trac.Frame.SprkOffVer.PivotFra  axle_y=Trac.Frame.SprkOffVer.Axle  idlerArm_y=Trac.Frame.SprkOffVer.IdlerArm  frame_mass=Trac.Frame.TrackFrame.Mass  frame_cg_offset=Trac.Frame.TrackFrame.CG  frame_moi=Trac.Frame.TrackFrame.MOI  frame_poi=Trac.Frame.TrackFrame.POI  frame_roller_cg_offset=Trac.Frame.SprkFrame.CG  frame_roller_mass=Trac.Frame.SprkFrame.Mass  frame_roller_moi=Trac.Frame.SprkFrame.MOI  frame_roller_poi=Trac.Frame.SprkFrame.POI  frame_susp_offset=Trac.Frame.SuspOffset  roller_frame_pivot_range=Trac.Frame.PivotFra.Range  roller_frame_pivot_k=Trac.Frame.PivotFra.LimitK  roller_frame_pivot_b=Trac.Frame.PivotFra.LimitB  roller_frame_pivot_tw=Trac.Frame.PivotFra.LimitTW  sprk_rolling_rad=Trac.Sprocket.ground_contact.rolling_radius  roller_lower_rolling_rad=Trac.Roller.Lower.ground_contact.rolling_radius  idlerF_rolling_rad=Trac.IdlerF.ground_contact.rolling_radius  idlerR_rolling_rad=Trac.IdlerR.ground_contact.rolling_radius  rolling_cyl_len=Trac.Belt.w  accent_vis_lext=1e-3  roller_lower_cyl_clr=Trac.Roller.Lower.clr  roller_lower_cyl_opc=Trac.Roller.Lower.opc  idlerR_rollvervis_clr=Trac.IdlerR.clr  idlerF_rollvervis_clr=Trac.IdlerF.clr  idlerR_rollervis_opc=Trac.IdlerR.opc  idlerF_rollervis_opc=Trac.IdlerF.opc  accMn=0.65  accMx=0.75  acc_clr=[0.8 0.8 0.8]  acc_opc=1  track_m=Trac.Vis.Track.m  track_cg_offset=Trac.Vis.Track.cg  track_moi=Trac.Vis.Track.moi  track_poi=Trac.Vis.Track.poi  track_xc=Trac.Vis.Track.track_xc  track_clr=Trac.Vis.Track.clr  track_opc=Trac.Vis.Track.opc  popup_sense_roller=Actuator Torque
      settings: AttributesFormatString=%<popup_trackFrame>
  Track RL : sm_rollerV_lib_lower_frame_idlerArm_i2u0l3/Track Contact Roller  sprk_wid_roll=Trac.Sprocket.Roller.wid  sprk_rad_roll=Trac.Sprocket.Roller.rad  sprk_clr=Trac.Sprocket.Roller.clr  sprk_opc=Trac.Sprocket.Roller.opc  sprk_rad_pitch=Trac.Sprocket.Spoke.pitch_rad  sprk_spoke_rad=Trac.Sprocket.Spoke.rad  sprk_spoke_num=Trac.Sprocket.nSpokes  sprk_spoke_len=Trac.Sprocket.Spoke.len  sprk_rim_spoke_xc=Trac.Sprocket.Rim.spoke_xc  sprk_rim_ir=Trac.Sprocket.Rim.rad_inner  sprk_rim_thk=Trac.Sprocket.Rim.thk  idlerR_rad=Trac.IdlerR.rad  idlerF_rad=Trac.IdlerF.rad  idlerR_total_len=Trac.IdlerR.len_total  idlerF_total_len=Trac.IdlerF.len_total  idlerR_avg_rho=Trac.IdlerR.rho_avg  idlerF_avg_rho=Trac.IdlerF.rho_avg  idlerR_clr=Trac.IdlerR.clr  idlerF_clr=Trac.IdlerF.clr  idlerR_opc=Trac.IdlerR.opc  idlerF_opc=Trac.IdlerF.opc  idlerR_contgeo_ptcld=Trac.IdlerR.ground_contact.ptcld.pts  idlerF_contgeo_ptcld=Trac.IdlerF.ground_contact.ptcld.pts  idlerR_contgeo_rad=Trac.IdlerR.ground_contact.ptcld.rad  idlerF_contgeo_rad=Trac.IdlerF.ground_contact.ptcld.rad  idlerR_contgeo_clr=Trac.IdlerR.belt_contact.clr  idlerF_contgeo_clr=Trac.IdlerF.belt_contact.clr  idlerR_contgeo_opc=Trac.IdlerR.belt_contact.opc  idlerF_contgeo_opc=Trac.IdlerF.belt_contact.opc  arm_idlerc=Trac.IdlerArm.Pivot_to_Idler  arm_tens_x=Trac.IdlerArm.Pivot_to_TensionerX  arm_tens_y=Trac.IdlerArm.Pivot_to_TensionerY  arm_wid=Trac.IdlerArm.wid  arm_thk=Trac.IdlerArm.thk  arm_rho=Trac.IdlerArm.rho  arm_clr=Trac.IdlerArm.clr  arm_opc=Trac.IdlerArm.opc  roller_lower_rad=Trac.Roller.Lower.rad  roller_lower_len=Trac.Roller.Lower.len  roller_lower_rho=Trac.Roller.Lower.rho  roller_lower_clr=Trac.Roller.Lower.clr  roller_lower_opc=Trac.Roller.Lower.opc  roller_lower_contgeo_ptcld=Trac.Roller.Lower.ground_contact.ptcld.pts  roller_lower_contgeo_rad=Trac.Roller.Lower.ground_contact.ptcld.rad  roller_lower_contgeo_clr=Trac.Roller.Lower.belt_contact.clr  roller_lower_contgeo_opc=Trac.Roller.Lower.belt_contact.opc  tensioner_cyl_len=Trac.IdlerF.Tensioner.cyl.len  tensioner_cyl_rad=Trac.IdlerF.Tensioner.cyl.rad  tensioner_cyl_rho=Trac.IdlerF.Tensioner.cyl.rho  tensioner_cyl_clr=Trac.IdlerF.Tensioner.cyl.clr  tensioner_cyl_opc=Trac.IdlerF.Tensioner.cyl.opc  tensioner_pist_len=Trac.IdlerF.Tensioner.piston.len  tensioner_pist_rad=Trac.IdlerF.Tensioner.piston.rad  tensioner_pist_rho=Trac.IdlerF.Tensioner.piston.rho  tensioner_pist_clr=Trac.IdlerF.Tensioner.piston.clr  tensioner_pist_opc=Trac.IdlerF.Tensioner.piston.opc  tensioner_br_len=Trac.IdlerF.Tensioner.bracket.len  tensioner_br_width=Trac.IdlerF.Tensioner.bracket.wid  tensioner_br_height=Trac.IdlerF.Tensioner.bracket.height  tensioner_br_thk=Trac.IdlerF.Tensioner.bracket.thk  tensioner_br_rho=Trac.IdlerF.Tensioner.bracket.rho  tensioner_br_clr=Trac.IdlerF.Tensioner.bracket.clr  tensioner_br_opc=Trac.IdlerF.Tensioner.bracket.opc  tensioner_eqpos=Trac.IdlerF.Tensioner.xeq  tensioner_x0=Trac.IdlerF.Tensioner.x0  tensioner_k=Trac.IdlerF.Tensioner.K  tensioner_b=Trac.IdlerF.Tensioner.B  popup_leftOrRight=Left  popup_trackFrame=Fixed  roller_lower_x=Trac.Frame.SprkOffLon.Lower  idlerFix_x=Trac.Frame.SprkOffLon.IdlerR  idlerArm_x=Trac.Frame.SprkOffLon.IdlerArm  tensionC_x=Trac.Frame.SprkOffLon.TensionC  frame_pivot_x=Trac.Frame.SprkOffLon.PivotFra  axle_x=Trac.Frame.SprkOffLon.Axle  roller_lower_y=Trac.Frame.SprkOffVer.Lower  idlerFix_y=Trac.Frame.SprkOffVer.IdlerR  tensionC_y=Trac.Frame.SprkOffVer.TensionC  frame_pivot_y=Trac.Frame.SprkOffVer.PivotFra  axle_y=Trac.Frame.SprkOffVer.Axle  idlerArm_y=Trac.Frame.SprkOffVer.IdlerArm  frame_mass=Trac.Frame.TrackFrame.Mass  frame_cg_offset=Trac.Frame.TrackFrame.CG  frame_moi=Trac.Frame.TrackFrame.MOI  frame_poi=Trac.Frame.TrackFrame.POI  frame_roller_cg_offset=Trac.Frame.SprkFrame.CG  frame_roller_mass=Trac.Frame.SprkFrame.Mass  frame_roller_moi=Trac.Frame.SprkFrame.MOI  frame_roller_poi=Trac.Frame.SprkFrame.POI  frame_susp_offset=Trac.Frame.SuspOffset  roller_frame_pivot_range=Trac.Frame.PivotFra.Range  roller_frame_pivot_k=Trac.Frame.PivotFra.LimitK  roller_frame_pivot_b=Trac.Frame.PivotFra.LimitB  roller_frame_pivot_tw=Trac.Frame.PivotFra.LimitTW  sprk_rolling_rad=Trac.Sprocket.ground_contact.rolling_radius  roller_lower_rolling_rad=Trac.Roller.Lower.ground_contact.rolling_radius  idlerF_rolling_rad=Trac.IdlerF.ground_contact.rolling_radius  idlerR_rolling_rad=Trac.IdlerR.ground_contact.rolling_radius  rolling_cyl_len=Trac.Belt.w  accent_vis_lext=1e-3  roller_lower_cyl_clr=Trac.Roller.Lower.clr  roller_lower_cyl_opc=Trac.Roller.Lower.opc  idlerR_rollvervis_clr=Trac.IdlerR.clr  idlerF_rollvervis_clr=Trac.IdlerF.clr  idlerR_rollervis_opc=Trac.IdlerR.opc  idlerF_rollervis_opc=Trac.IdlerF.opc  accMn=0.65  accMx=0.75  acc_clr=[0.8 0.8 0.8]  acc_opc=1  track_m=Trac.Vis.Track.m  track_cg_offset=Trac.Vis.Track.cg  track_moi=Trac.Vis.Track.moi  track_poi=Trac.Vis.Track.poi  track_xc=Trac.Vis.Track.track_xc  track_clr=Trac.Vis.Track.clr  track_opc=Trac.Vis.Track.opc  popup_sense_roller=Actuator Torque
      settings: AttributesFormatString=%<popup_trackFrame>
  Track RR : sm_rollerV_lib_lower_frame_idlerArm_i2u0l3/Track Contact Roller  sprk_wid_roll=Trac.Sprocket.Roller.wid  sprk_rad_roll=Trac.Sprocket.Roller.rad  sprk_clr=Trac.Sprocket.Roller.clr  sprk_opc=Trac.Sprocket.Roller.opc  sprk_rad_pitch=Trac.Sprocket.Spoke.pitch_rad  sprk_spoke_rad=Trac.Sprocket.Spoke.rad  sprk_spoke_num=Trac.Sprocket.nSpokes  sprk_spoke_len=Trac.Sprocket.Spoke.len  sprk_rim_spoke_xc=Trac.Sprocket.Rim.spoke_xc  sprk_rim_ir=Trac.Sprocket.Rim.rad_inner  sprk_rim_thk=Trac.Sprocket.Rim.thk  idlerR_rad=Trac.IdlerR.rad  idlerF_rad=Trac.IdlerF.rad  idlerR_total_len=Trac.IdlerR.len_total  idlerF_total_len=Trac.IdlerF.len_total  idlerR_avg_rho=Trac.IdlerR.rho_avg  idlerF_avg_rho=Trac.IdlerF.rho_avg  idlerR_clr=Trac.IdlerR.clr  idlerF_clr=Trac.IdlerF.clr  idlerR_opc=Trac.IdlerR.opc  idlerF_opc=Trac.IdlerF.opc  idlerR_contgeo_ptcld=Trac.IdlerR.ground_contact.ptcld.pts  idlerF_contgeo_ptcld=Trac.IdlerF.ground_contact.ptcld.pts  idlerR_contgeo_rad=Trac.IdlerR.ground_contact.ptcld.rad  idlerF_contgeo_rad=Trac.IdlerF.ground_contact.ptcld.rad  idlerR_contgeo_clr=Trac.IdlerR.belt_contact.clr  idlerF_contgeo_clr=Trac.IdlerF.belt_contact.clr  idlerR_contgeo_opc=Trac.IdlerR.belt_contact.opc  idlerF_contgeo_opc=Trac.IdlerF.belt_contact.opc  arm_idlerc=Trac.IdlerArm.Pivot_to_Idler  arm_tens_x=Trac.IdlerArm.Pivot_to_TensionerX  arm_tens_y=Trac.IdlerArm.Pivot_to_TensionerY  arm_wid=Trac.IdlerArm.wid  arm_thk=Trac.IdlerArm.thk  arm_rho=Trac.IdlerArm.rho  arm_clr=Trac.IdlerArm.clr  arm_opc=Trac.IdlerArm.opc  roller_lower_rad=Trac.Roller.Lower.rad  roller_lower_len=Trac.Roller.Lower.len  roller_lower_rho=Trac.Roller.Lower.rho  roller_lower_clr=Trac.Roller.Lower.clr  roller_lower_opc=Trac.Roller.Lower.opc  roller_lower_contgeo_ptcld=Trac.Roller.Lower.ground_contact.ptcld.pts  roller_lower_contgeo_rad=Trac.Roller.Lower.ground_contact.ptcld.rad  roller_lower_contgeo_clr=Trac.Roller.Lower.belt_contact.clr  roller_lower_contgeo_opc=Trac.Roller.Lower.belt_contact.opc  tensioner_cyl_len=Trac.IdlerF.Tensioner.cyl.len  tensioner_cyl_rad=Trac.IdlerF.Tensioner.cyl.rad  tensioner_cyl_rho=Trac.IdlerF.Tensioner.cyl.rho  tensioner_cyl_clr=Trac.IdlerF.Tensioner.cyl.clr  tensioner_cyl_opc=Trac.IdlerF.Tensioner.cyl.opc  tensioner_pist_len=Trac.IdlerF.Tensioner.piston.len  tensioner_pist_rad=Trac.IdlerF.Tensioner.piston.rad  tensioner_pist_rho=Trac.IdlerF.Tensioner.piston.rho  tensioner_pist_clr=Trac.IdlerF.Tensioner.piston.clr  tensioner_pist_opc=Trac.IdlerF.Tensioner.piston.opc  tensioner_br_len=Trac.IdlerF.Tensioner.bracket.len  tensioner_br_width=Trac.IdlerF.Tensioner.bracket.wid  tensioner_br_height=Trac.IdlerF.Tensioner.bracket.height  tensioner_br_thk=Trac.IdlerF.Tensioner.bracket.thk  tensioner_br_rho=Trac.IdlerF.Tensioner.bracket.rho  tensioner_br_clr=Trac.IdlerF.Tensioner.bracket.clr  tensioner_br_opc=Trac.IdlerF.Tensioner.bracket.opc  tensioner_eqpos=Trac.IdlerF.Tensioner.xeq  tensioner_x0=Trac.IdlerF.Tensioner.x0  tensioner_k=Trac.IdlerF.Tensioner.K  tensioner_b=Trac.IdlerF.Tensioner.B  popup_leftOrRight=Right  popup_trackFrame=Fixed  roller_lower_x=Trac.Frame.SprkOffLon.Lower  idlerFix_x=Trac.Frame.SprkOffLon.IdlerR  idlerArm_x=Trac.Frame.SprkOffLon.IdlerArm  tensionC_x=Trac.Frame.SprkOffLon.TensionC  frame_pivot_x=Trac.Frame.SprkOffLon.PivotFra  axle_x=Trac.Frame.SprkOffLon.Axle  roller_lower_y=Trac.Frame.SprkOffVer.Lower  idlerFix_y=Trac.Frame.SprkOffVer.IdlerR  tensionC_y=Trac.Frame.SprkOffVer.TensionC  frame_pivot_y=Trac.Frame.SprkOffVer.PivotFra  axle_y=Trac.Frame.SprkOffVer.Axle  idlerArm_y=Trac.Frame.SprkOffVer.IdlerArm  frame_mass=Trac.Frame.TrackFrame.Mass  frame_cg_offset=Trac.Frame.TrackFrame.CG  frame_moi=Trac.Frame.TrackFrame.MOI  frame_poi=Trac.Frame.TrackFrame.POI  frame_roller_cg_offset=Trac.Frame.SprkFrame.CG  frame_roller_mass=Trac.Frame.SprkFrame.Mass  frame_roller_moi=Trac.Frame.SprkFrame.MOI  frame_roller_poi=Trac.Frame.SprkFrame.POI  frame_susp_offset=Trac.Frame.SuspOffset  roller_frame_pivot_range=Trac.Frame.PivotFra.Range  roller_frame_pivot_k=Trac.Frame.PivotFra.LimitK  roller_frame_pivot_b=Trac.Frame.PivotFra.LimitB  roller_frame_pivot_tw=Trac.Frame.PivotFra.LimitTW  sprk_rolling_rad=Trac.Sprocket.ground_contact.rolling_radius  roller_lower_rolling_rad=Trac.Roller.Lower.ground_contact.rolling_radius  idlerF_rolling_rad=Trac.IdlerF.ground_contact.rolling_radius  idlerR_rolling_rad=Trac.IdlerR.ground_contact.rolling_radius  rolling_cyl_len=Trac.Belt.w  accent_vis_lext=1e-3  roller_lower_cyl_clr=Trac.Roller.Lower.clr  roller_lower_cyl_opc=Trac.Roller.Lower.opc  idlerR_rollvervis_clr=Trac.IdlerR.clr  idlerF_rollvervis_clr=Trac.IdlerF.clr  idlerR_rollervis_opc=Trac.IdlerR.opc  idlerF_rollervis_opc=Trac.IdlerF.opc  accMn=0.65  accMx=0.75  acc_clr=[0.8 0.8 0.8]  acc_opc=1  track_m=Trac.Vis.Track.m  track_cg_offset=Trac.Vis.Track.cg  track_moi=Trac.Vis.Track.moi  track_poi=Trac.Vis.Track.poi  track_xc=Trac.Vis.Track.track_xc  track_clr=Trac.Vis.Track.clr  track_opc=Trac.Vis.Track.opc  popup_sense_roller=Actuator Torque
      settings: AttributesFormatString=%<popup_trackFrame>
  Vehicle Speed : Subsystem  Variant=on  VariantControlMode=label  VariantControl=Choice  LabelModeActiveChoice=Fwd
      settings: AttributesFormatString=%<LabelModeActiveChoice>
      mask Display: disp(' ')
  wires:
  Track RL/1 -> [mRL]
  Body Sensor/1 -> [B]
  Vehicle Speed/1(wL) -> Steering/1
  [B] -> Scopes/1(Body)  "Body"
  [mRR] -> Scopes/5(RR)  "Track RR"
  [mRL] -> Scopes/4(RL)  "Track RL"
  Track RR/1 -> [mRR]
  Steer Angle/1 -> Steer On/1
  Steering/3 -> [wFR]
  Steering/2 -> [wFL]
  [wFR] -> Simulink-PS Converter3/1
  [wFL] -> Simulink-PS Converter2/1
  Steering/1 -> [wRL]
  Steering/4 -> [wRR]
  [wRR] -> Simulink-PS Converter1/1
  [wRL] -> Simulink-PS Converter/1
  Steering/5 -> Terminator/1
  Track FR/1 -> [mFR]
  Track FL/1 -> [mFL]
  [mFL] -> Scopes/2(FL)  "Track FL"
  [mFR] -> Scopes/3(FR)  "Track FR"
  Steer On/1 -> Steering/2
  connections:
  Chassis/RConn2 -- Track RR/LConn2
  Chassis/LConn2 -- Track RL/LConn2
  Assembly to World/RConn1 -- Body Sensor/LConn1 -- Chassis/RConn3
  Track RL/RConn1 -- Connection Label/LConn1
  Track RR/RConn1 -- Connection Label2/LConn1
  Simulink-PS Converter1/RConn1 -- Angular Velocity Source RR/RConn1
  Angular Velocity Source RR/RConn2 -- MRRef RR/LConn1
  Track RL/RConn2 -- Drive Shaft RL/RConn1
  Drive Shaft RR/LConn1 -- Angular Velocity Source RR/LConn1
  Track RR/RConn2 -- Drive Shaft RR/RConn1
  Simulink-PS Converter/RConn1 -- Angular Velocity Source RL/RConn1
  Angular Velocity Source RL/RConn2 -- MRRef RL/LConn1
  Drive Shaft RL/LConn1 -- Angular Velocity Source RL/LConn1
  Config/LConn1 -- Assembly to World/LConn1 -- Scene/RConn1
  Scene/LConn1 -- Connection Label1/LConn1
  Scene/LConn2 -- Connection Label3/LConn1
  Connection Label4/LConn1 -- Scene/LConn3
  Connection Label5/LConn1 -- Scene/LConn4
  Str FL/LConn1 -- Chassis/LConn1
  Angular Velocity Source FL/RConn2 -- MRRef FL/LConn1
  Simulink-PS Converter2/RConn1 -- Angular Velocity Source FL/RConn1
  Track FL/RConn2 -- Drive Shaft FL/RConn1
  Drive Shaft FL/LConn1 -- Angular Velocity Source FL/LConn1
  Track FR/RConn2 -- Drive Shaft FR/RConn1
  Drive Shaft FR/LConn1 -- Angular Velocity Source FR/LConn1
  Angular Velocity Source FR/RConn2 -- MRRef FR/LConn1
  Simulink-PS Converter3/RConn1 -- Angular Velocity Source FR/RConn1
  Connection Label6/LConn1 -- Track FR/RConn1
  Connection Label7/LConn1 -- Track FL/RConn1
  Str FR/LConn1 -- Chassis/RConn1
  Str FR/RConn1 -- Track FR/LConn2
  Str FL/RConn1 -- Track FL/LConn2
  Steering/LConn1 -- Str FL/LConn2
  Steering/RConn1 -- Str FR/LConn2

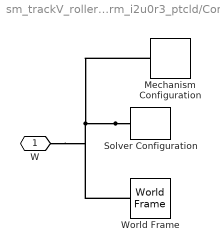
== system sm_trackV_roller4_IdlerArm_i2u0r3_ptcld/Config ==
  Mechanism Configuration : sm_lib/Utilities/Mechanism Configuration  UniformGravity=Constant  GravityVector=[0 0 -9.80665]  GravityVectorUnits=m/s^2  LinearizationDelta=0.001  JointModeTransitionNonlinearIterations=2
  Solver Configuration : nesl_utility/Solver Configuration  PhysicalDomain=network_engine_domain  SubClassName=solver  LeftPortType=input  RightPortType=generic  Tones=[]  Harmonics=[]  SimulateNoise=off  Profile=off  UseLocalSampling=off  EnableSwitchedLinearOptims=on  FrequencyDomain=off  UseCCode=off  RelTol=0.001  AbsTol=1e-06  MinStep=1e-09  ToWorkspace=off  RevertToSquareIcSolve=off  NumHomotopyIterations=100  PhasorMode=off  PhasorModeNumHarmonics=1  ConsistencySolver=NEWTON_XTOL_AFTER_FTOL  CanonicalOrdering=UNORDERED  OptimizeIntermediates=UNOPTIMIZED  IndexReductionMethod=DerivativeReplacement  DoDC=off  ResidualTolerance=1e-09  ConsistencyTolSource=GLOBAL  ConsistencyAbsTol=0.001  ConsistencyRelTol=0.001  ConsistencyTolFactor=0.001  UseLocalSolver=off  LocalSolverChoice=NE_BACKWARD_EULER_ADVANCER  ResolveIndetEquations=on  FunctionEvalNumThread=1  LocalSolverSampleTime=0.001  DoFixedCost=off  MaxNonlinIter=3  MaxModeIter=2  ComputeImpulses=off  ImpulseIterations=2  LinearAlgebra=Sparse  LinearAlgebraNumThread=0  EquationFormulation=NE_TIME_EF  DelaysMemoryBudget=1024  AutomaticFiltering=on  FilteringTimeConstant=0.001  PartitionStorageMethod=AS_NEEDED  PartitionMemoryBudget=1024  PartitionMethod=FAST  MultibodyUseLocalSolver=off  MultibodyLocalSolverChoice=ODE1  MultibodyLocalSolverSampleTime=0.001
  World Frame : sm_lib/Frames and Transforms/World Frame
  W : PMIOPort  Side=Left
  connections:
  Solver Configuration/RConn1 -- Mechanism Configuration/RConn1 -- W/RConn1 -- World Frame/RConn1
